simulink model "PlatoonController"  (R2018a)
settings: Solver=FixedStepDiscrete  StartTime=0.0  StopTime=2  MaxStep=0.01  RelTol=1e-4
settings Model: Creator=ATRC237_GUO  LastModifiedBy=ATRC237_GUO
settings DataIOCC: LimitDataPoints=on  SaveOutput=off  SaveTime=off
settings OptimizationCC: DefaultParameterBehavior=Inlined  UseDivisionForNetSlopeComputation=on  UseFloatMulNetSlope=on  InlineInvariantSignals=on  PassReuseOutputArgsAs=Individual arguments  ExpressionDepthLimit=2147483647  ZeroExternalMemoryAtStartup=off  ZeroInternalMemoryAtStartup=off  NoFixptDivByZeroProtection=on  EfficientFloat2IntCast=on  LifeSpan=1  OptimizeBlockOrder=speed  DifferentSizesBufferReuse=on
settings DebuggingCC: UnderspecifiedInitializationDetection=Classic  MergeDetectMultiDrivingBlocksExec=none  ParameterTunabilityLossMsg=error  FcnCallInpInsideContextMsg=warning  AllowSymbolicDim=off  StateNameClashWarn=warning  SFUnexpectedBacktrackingDiag=warning  SFNoUnconditionalDefaultTransitionDiag=warning  SFExecutionAtInitializationDiag=none
settings HardwareCC: ProdLongLongMode=on
settings SFSimCC: MATLABDynamicMemAlloc=off
settings RTWCC: SystemTargetFile=ert.tlc  TemplateMakefile=ert_default_tmf  GenerateReport=on  IncludeHyperlinkInReport=on  LaunchReport=on  TargetLang=C++  GenerateTraceInfo=on  GenerateTraceReport=on  GenerateTraceReportSl=on  GenerateTraceReportSf=on  GenerateTraceReportEml=on
settings CodeAppCC: ForceParamTrailComments=on  IgnoreCustomStorageClasses=off  OperatorAnnotations=on  SimulinkDataObjDesc=on  SFDataObjDesc=on  CustomSymbolStrGlobalVar=rt$N$M  CustomSymbolStrType=$N$M  CustomSymbolStrFcn=$N$M$F  CustomSymbolStrMacro=$N$M  InsertBlockDesc=on
settings ERTTargetCC: TargetLangStandard=C++03 (ISO)  GenerateSampleERTMain=on  IncludeMdlTerminateFcn=off  CombineSignalStateStructs=on  MultiInstanceERTCode=on  CodeInterfacePackaging=C++ class  SupportComplex=off  SupportContinuousTime=on  InlinedParameterPlacement=NonHierarchical  RootIOFormat=Structure reference  ERTCustomFileTemplate=example_file_process.tlc  ERTFilePackagingFormat=CompactWithDataFile

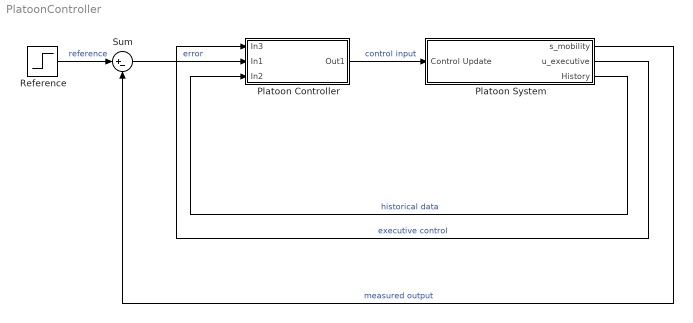
== system PlatoonController ==
  Platoon Controller : Subsystem
  Platoon System : Subsystem
  Reference : Step  SampleTime=0
  Sum : Sum  Inputs=|+-
  wires:
  Reference/1 -> Sum/1  "reference"
  Platoon System/1(s_mobility) -> Sum/2  "measured output"
  Platoon Controller/1(Out1) -> Platoon System/1(Control Update)  "control input"
  Platoon System/3(History) -> Platoon Controller/3(In2)  "historical data"
  Sum/1 -> Platoon Controller/2(In1)  "error"
  Platoon System/2(u_executive) -> Platoon Controller/1(In3)  "executive control"

== system PlatoonController/Platoon Controller ==
  In3 : Inport
  In1 : Inport  Port=2
  In2 : Inport  Port=3
  HLC : Subsystem
  LLC : Subsystem
  PLC : Subsystem
  Out1 : Outport
  wires:
  HLC/1(Out1) -> LLC/1(In1)
  PLC/1(Out1) -> HLC/1(In1)
  In1/1 -> PLC/2(Current)
  LLC/1(Out1) -> Out1/1
  In2/1 -> PLC/3(History)
  In3/1 -> PLC/1(Executive)

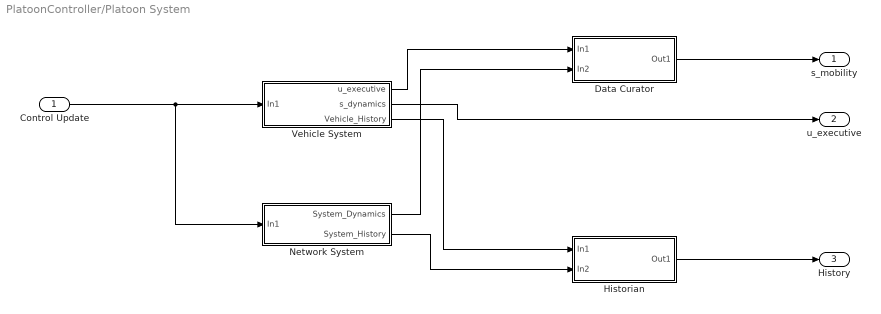
== system PlatoonController/Platoon System ==
  Control Update : Inport
  Data Curator : Subsystem
  Historian : Subsystem
  Network System : Subsystem
  Vehicle System : Subsystem
  s_mobility : Outport
  u_executive : Outport  Port=2
  History : Outport  Port=3
  wires:
  Control Update/1 -> Network System/1(In1), Vehicle System/1(In1)
  Historian/1(Out1) -> History/1
  Data Curator/1(Out1) -> s_mobility/1
  Vehicle System/1(u_executive) -> Data Curator/1(In1)
  Vehicle System/3(Vehicle_History) -> Historian/1(In1)
  Network System/1(System_Dynamics) -> Data Curator/2(In2)
  Network System/2(System_History) -> Historian/2(In2)
  Vehicle System/2(s_dynamics) -> u_executive/1

== system PlatoonController/Platoon Controller/HLC ==
  In1 : Inport
  Lateral Control : Subsystem
  Longitudinal Control : Subsystem
  Maneuver Converter : Subsystem
  Vector Concatenate : Concatenate
  Out1 : Outport
  wires:
  Longitudinal Control/1("u_accel ") -> Vector Concatenate/1
  Vector Concatenate/1 -> Out1/1
  Lateral Control/1(u_steer) -> Vector Concatenate/2
  In1/1 -> Maneuver Converter/1(In1)
  Maneuver Converter/1(Out1) -> Longitudinal Control/1(In1)
  Maneuver Converter/2(Out2) -> Lateral Control/1(In1)

== system PlatoonController/Platoon Controller/LLC ==
  In1 : Inport
  Brake : Subsystem
  Output State : Subsystem
  Steering Wheel : Subsystem
  Throttle : Subsystem
  Out1 : Outport
  wires:
  In1/1 -> Throttle/1(In1), Brake/1(In1), Steering Wheel/1(In1)
  Output State/1(Out1) -> Out1/1
  Throttle/1(Out1) -> Output State/1(In3)
  Brake/1(Out1) -> Output State/2(In1)
  Steering Wheel/1(Out1) -> Output State/3(In2)

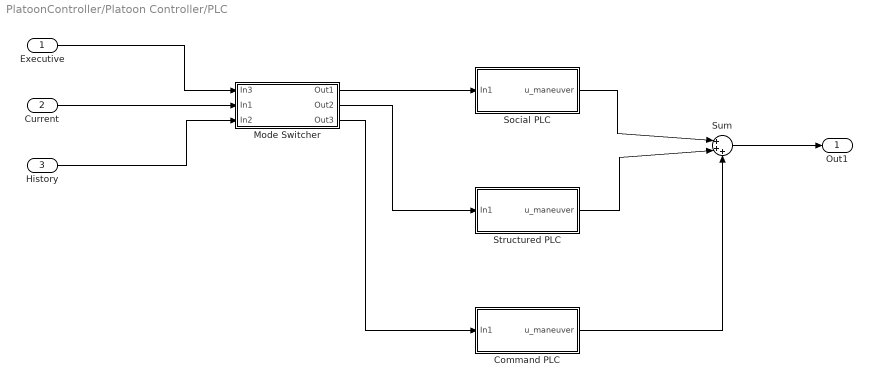
== system PlatoonController/Platoon Controller/PLC ==
  Executive : Inport
  Current : Inport  Port=2
  History : Inport  Port=3
  Command PLC : Subsystem
  Mode Switcher : Subsystem
  Social PLC : Subsystem
  Structured PLC : Subsystem
  Sum : Sum  Inputs=|+++
  Out1 : Outport
  wires:
  Current/1 -> Mode Switcher/2(In1)
  Mode Switcher/1(Out1) -> Social PLC/1(In1)
  Mode Switcher/2(Out2) -> Structured PLC/1(In1)
  Social PLC/1(u_maneuver) -> Sum/1
  Structured PLC/1(u_maneuver) -> Sum/2
  Sum/1 -> Out1/1
  History/1 -> Mode Switcher/3(In2)
  Executive/1 -> Mode Switcher/1(In3)
  Command PLC/1(u_maneuver) -> Sum/3
  Mode Switcher/3(Out3) -> Command PLC/1(In1)

== system PlatoonController/Platoon System/Data Curator ==
  In1 : Inport
  In2 : Inport  Port=2
  Vector Concatenate : Concatenate
  Out1 : Outport
  wires:
  In2/1 -> Vector Concatenate/2
  In1/1 -> Vector Concatenate/1
  Vector Concatenate/1 -> Out1/1

== system PlatoonController/Platoon System/Historian ==
  In1 : Inport
  In2 : Inport  Port=2
  Vector Concatenate : Concatenate
  Out1 : Outport
  wires:
  In1/1 -> Vector Concatenate/1
  In2/1 -> Vector Concatenate/2
  Vector Concatenate/1 -> Out1/1

== system PlatoonController/Platoon System/Network System ==
  In1 : Inport
  CAV Network System : Subsystem
  Communication System : Subsystem
  Storage System : Subsystem
  System_Dynamics : Outport
  System_History : Outport  Port=2
  wires:
  Communication System/1(Out1) -> CAV Network System/1(In1)
  CAV Network System/1(Out1) -> System_Dynamics/1, Storage System/1(In1)
  In1/1 -> Communication System/1(In1)
  Storage System/1(Out1) -> System_History/1

== system PlatoonController/Platoon System/Vehicle System ==
  In1 : Inport
  CAV System : Subsystem
  Storage System : Subsystem
  u_executive : Outport
  s_dynamics : Outport  Port=2
  Vehicle_History : Outport  Port=3
  wires:
  In1/1 -> Storage System/1(In1), CAV System/1(In1)
  CAV System/1(u_executive) -> u_executive/1
  Storage System/1(Out1) -> Vehicle_History/1
  CAV System/2(s_dynamics) -> s_dynamics/1

== system PlatoonController/Platoon Controller/HLC/Lateral Control ==
  In1 : Inport
  "Steer " : Subsystem
  u_steer : Outport
  wires:
  In1/1 -> "Steer "/1(In1)
  "Steer "/1(Out1) -> u_steer/1

== system PlatoonController/Platoon Controller/HLC/Longitudinal Control ==
  In1 : Inport
  Acceleration : Subsystem
  Brake : Subsystem
  Throttle : Subsystem
  "u_accel " : Outport
  wires:
  Throttle/1(Out1) -> Acceleration/1(In1)
  Brake/1(Out1) -> Acceleration/2(In2)
  Acceleration/1(Out1) -> "u_accel "/1
  In1/1 -> Brake/1(In1), Throttle/1(In1)

== system PlatoonController/Platoon Controller/HLC/Maneuver Converter ==
  In1 : Inport
  Out1 : Outport
  Out2 : Outport  Port=2
  wires:
  In1/1 -> Out1/1

== system PlatoonController/Platoon Controller/LLC/Brake ==
  In1 : Inport
  Out1 : Outport
  wires:
  In1/1 -> Out1/1

== system PlatoonController/Platoon Controller/LLC/Output State ==
  In3 : Inport
  In1 : Inport  Port=2
  In2 : Inport  Port=3
  Out1 : Outport
  wires:
  In1/1 -> Out1/1

== system PlatoonController/Platoon Controller/LLC/Steering Wheel ==
  In1 : Inport
  Out1 : Outport
  wires:
  In1/1 -> Out1/1

== system PlatoonController/Platoon Controller/LLC/Throttle ==
  In1 : Inport
  Out1 : Outport
  wires:
  In1/1 -> Out1/1

== system PlatoonController/Platoon Controller/PLC/Command PLC ==
  In1 : Inport
  Maneuver Calculator : Subsystem
  Predictor : Subsystem
  Recognizer : Subsystem
  Sustainer : Subsystem
  Vector Concatenate : Concatenate
  u_maneuver : Outport
  wires:
  Sustainer/1(Out1) -> Maneuver Calculator/1(In1), Predictor/1(In1)
  Recognizer/1(Out1) -> Vector Concatenate/1, Sustainer/1(In1)
  Predictor/1(Out1) -> Maneuver Calculator/2(In2)
  Maneuver Calculator/1(Maneuver_Coefficient) -> Vector Concatenate/2
  In1/1 -> Recognizer/1(In1)
  Vector Concatenate/1 -> u_maneuver/1

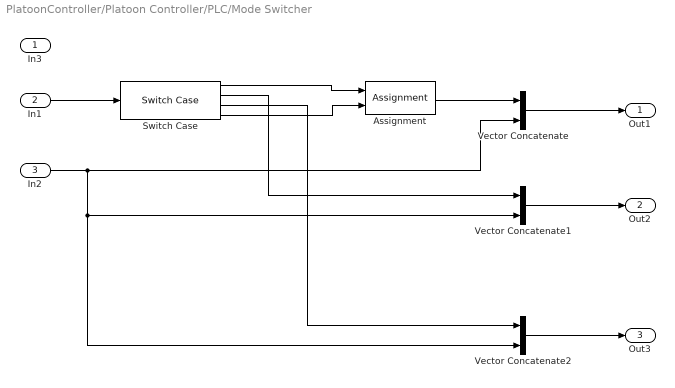
== system PlatoonController/Platoon Controller/PLC/Mode Switcher ==
  In3 : Inport
  In1 : Inport  Port=2
  In2 : Inport  Port=3
  Assignment : Assignment  DiagnosticForDimensions=Warning  IndexOptions=Index vector (dialog)  Indices=1  OutputSizes=1
  Switch Case : SwitchCase  CaseConditions={1, 2, 3}
  Vector Concatenate : Concatenate
  Vector Concatenate1 : Concatenate
  Vector Concatenate2 : Concatenate
  Out1 : Outport
  Out2 : Outport  Port=2
  Out3 : Outport  Port=3
  wires:
  In1/1 -> Switch Case/1
  Switch Case/1 -> Assignment/1
  Switch Case/4 -> Assignment/2
  Vector Concatenate1/1 -> Out2/1
  Assignment/1 -> Vector Concatenate/1
  Switch Case/2 -> Vector Concatenate1/1
  Vector Concatenate/1 -> Out1/1
  Vector Concatenate2/1 -> Out3/1
  In2/1 -> Vector Concatenate/2, Vector Concatenate2/2, Vector Concatenate1/2
  Switch Case/3 -> Vector Concatenate2/1

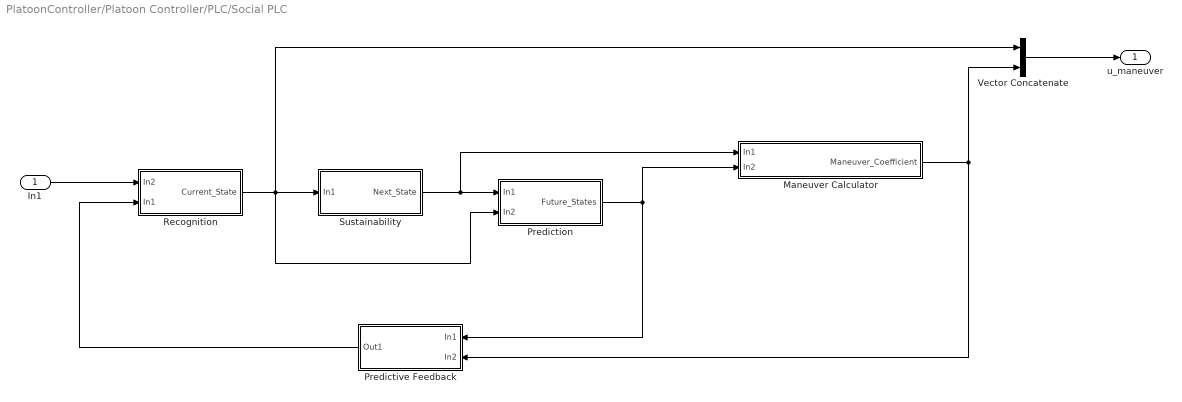
== system PlatoonController/Platoon Controller/PLC/Social PLC ==
  In1 : Inport
  Maneuver Calculator : Subsystem
  Prediction : Subsystem
  Predictive Feedback : Subsystem
  Recognition : Subsystem
  Sustainability : Subsystem
  Vector Concatenate : Concatenate
  u_maneuver : Outport
  wires:
  Prediction/1(Future_States) -> Maneuver Calculator/2(In2), Predictive Feedback/1(In1)
  In1/1 -> Recognition/1(In2)
  Sustainability/1(Next_State) -> Maneuver Calculator/1(In1), Prediction/1(In1)
  Recognition/1(Current_State) -> Vector Concatenate/1, Prediction/2(In2), Sustainability/1(In1)
  Maneuver Calculator/1(Maneuver_Coefficient) -> Vector Concatenate/2, Predictive Feedback/2(In2)
  Predictive Feedback/1(Out1) -> Recognition/2(In1)
  Vector Concatenate/1 -> u_maneuver/1

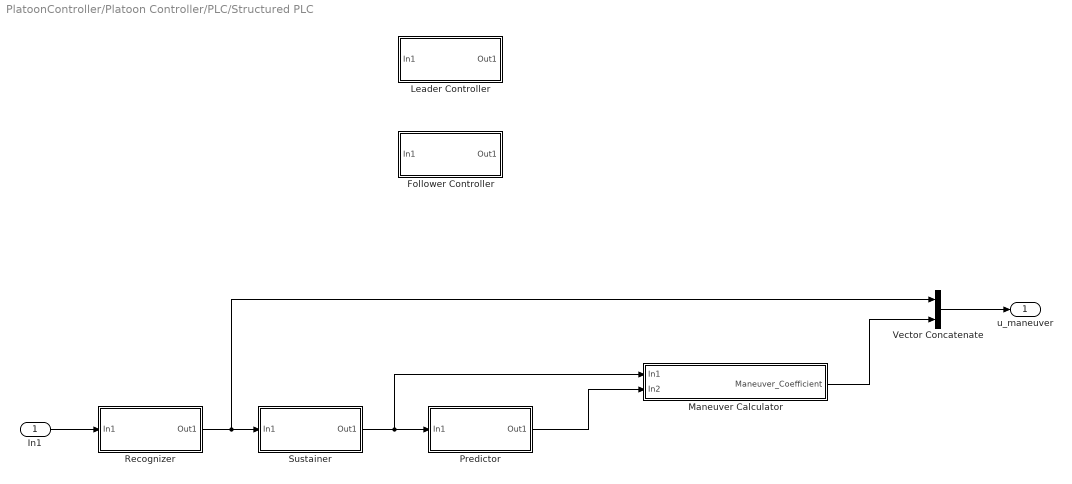
== system PlatoonController/Platoon Controller/PLC/Structured PLC ==
  In1 : Inport
  Follower Controller : Subsystem
  Leader Controller : Subsystem
  Maneuver Calculator : Subsystem
  Predictor : Subsystem
  Recognizer : Subsystem
  Sustainer : Subsystem
  Vector Concatenate : Concatenate
  u_maneuver : Outport
  wires:
  Sustainer/1(Out1) -> Maneuver Calculator/1(In1), Predictor/1(In1)
  Recognizer/1(Out1) -> Vector Concatenate/1, Sustainer/1(In1)
  Predictor/1(Out1) -> Maneuver Calculator/2(In2)
  Maneuver Calculator/1(Maneuver_Coefficient) -> Vector Concatenate/2
  In1/1 -> Recognizer/1(In1)
  Vector Concatenate/1 -> u_maneuver/1

== system PlatoonController/Platoon System/Network System/CAV Network System ==
  In1 : Inport
  Out1 : Outport
  wires:
  In1/1 -> Out1/1

== system PlatoonController/Platoon System/Network System/Communication System ==
  In1 : Inport
  Out1 : Outport
  wires:
  In1/1 -> Out1/1

== system PlatoonController/Platoon System/Network System/Storage System ==
  In1 : Inport
  Out1 : Outport
  wires:
  In1/1 -> Out1/1

== system PlatoonController/Platoon System/Vehicle System/CAV System ==
  In1 : Inport
  AVCB : Subsystem
  Vehicle Dynamics : Subsystem
  u_executive : Outport
  s_dynamics : Outport  Port=2
  wires:
  In1/1 -> AVCB/1(In1), Vehicle Dynamics/1(In1)
  AVCB/1(Out1) -> u_executive/1
  Vehicle Dynamics/1(Out1) -> s_dynamics/1

== system PlatoonController/Platoon System/Vehicle System/Storage System ==
  In1 : Inport
  Out1 : Outport
  wires:
  In1/1 -> Out1/1

== system PlatoonController/Platoon Controller/HLC/Lateral Control/Steer  ==
  In1 : Inport
  Out1 : Outport
  wires:
  In1/1 -> Out1/1

== system PlatoonController/Platoon Controller/HLC/Longitudinal Control/Acceleration ==
  In1 : Inport
  In2 : Inport  Port=2
  Out1 : Outport
  wires:
  In1/1 -> Out1/1

== system PlatoonController/Platoon Controller/HLC/Longitudinal Control/Brake ==
  In1 : Inport
  Out1 : Outport
  wires:
  In1/1 -> Out1/1

== system PlatoonController/Platoon Controller/HLC/Longitudinal Control/Throttle ==
  In1 : Inport
  Out1 : Outport
  wires:
  In1/1 -> Out1/1

== system PlatoonController/Platoon Controller/PLC/Command PLC/Maneuver Calculator ==
  In1 : Inport
  In2 : Inport  Port=2
  Sum : Sum  Inputs=|++
  Maneuver_Coefficient : Outport
  wires:
  In2/1 -> Sum/1
  In1/1 -> Sum/2
  Sum/1 -> Maneuver_Coefficient/1

== system PlatoonController/Platoon Controller/PLC/Command PLC/Predictor ==
  In1 : Inport
  Out1 : Outport
  wires:
  In1/1 -> Out1/1

== system PlatoonController/Platoon Controller/PLC/Command PLC/Recognizer ==
  In1 : Inport
  Out1 : Outport
  wires:
  In1/1 -> Out1/1

== system PlatoonController/Platoon Controller/PLC/Command PLC/Sustainer ==
  In1 : Inport
  Out1 : Outport
  wires:
  In1/1 -> Out1/1

== system PlatoonController/Platoon Controller/PLC/Social PLC/Maneuver Calculator ==
  In1 : Inport
  In2 : Inport  Port=2
  Sum : Sum  Inputs=|++
  Maneuver_Coefficient : Outport
  wires:
  In2/1 -> Sum/1
  In1/1 -> Sum/2
  Sum/1 -> Maneuver_Coefficient/1

== system PlatoonController/Platoon Controller/PLC/Social PLC/Prediction ==
  In1 : Inport
  In2 : Inport  Port=2
  Predictor : Subsystem
  Future_States : Outport
  wires:
  In1/1 -> Predictor/1(In1)
  Predictor/1(Out1) -> Future_States/1
  In2/1 -> Predictor/2(In2)

== system PlatoonController/Platoon Controller/PLC/Social PLC/Predictive Feedback ==
  In1 : Inport
  In2 : Inport  Port=2
  Vector Concatenate : Concatenate
  Out1 : Outport
  wires:
  In2/1 -> Vector Concatenate/2
  In1/1 -> Vector Concatenate/1
  Vector Concatenate/1 -> Out1/1

== system PlatoonController/Platoon Controller/PLC/Social PLC/Recognition ==
  In2 : Inport
  In1 : Inport  Port=2
  Estimator : Subsystem
  Refiner : Subsystem
  Current_State : Outport
  wires:
  In2/1 -> Estimator/1(In1)
  In1/1 -> Refiner/2(In2)
  Estimator/1(Out1) -> Refiner/1(In1)
  Refiner/1(Out1) -> Current_State/1

== system PlatoonController/Platoon Controller/PLC/Social PLC/Sustainability ==
  In1 : Inport
  Negotiator : Subsystem
  Optimizer : Subsystem
  Next_State : Outport
  wires:
  Optimizer/3(u_vehicle) -> Negotiator/3(In3)
  Optimizer/1(u_crowd) -> Negotiator/1(In1)
  Optimizer/2(u_safety) -> Negotiator/2(In2)
  In1/1 -> Optimizer/1(In1)
  Negotiator/1(Out1) -> Next_State/1

== system PlatoonController/Platoon Controller/PLC/Structured PLC/Follower Controller ==
  In1 : Inport
  Out1 : Outport
  wires:
  In1/1 -> Out1/1

== system PlatoonController/Platoon Controller/PLC/Structured PLC/Leader Controller ==
  In1 : Inport
  Out1 : Outport
  wires:
  In1/1 -> Out1/1

== system PlatoonController/Platoon Controller/PLC/Structured PLC/Maneuver Calculator ==
  In1 : Inport
  In2 : Inport  Port=2
  Sum : Sum  Inputs=|++
  Maneuver_Coefficient : Outport
  wires:
  In2/1 -> Sum/1
  In1/1 -> Sum/2
  Sum/1 -> Maneuver_Coefficient/1

== system PlatoonController/Platoon Controller/PLC/Structured PLC/Predictor ==
  In1 : Inport
  Out1 : Outport
  wires:
  In1/1 -> Out1/1

== system PlatoonController/Platoon Controller/PLC/Structured PLC/Recognizer ==
  In1 : Inport
  Out1 : Outport
  wires:
  In1/1 -> Out1/1

== system PlatoonController/Platoon Controller/PLC/Structured PLC/Sustainer ==
  In1 : Inport
  Out1 : Outport
  wires:
  In1/1 -> Out1/1

== system PlatoonController/Platoon System/Vehicle System/CAV System/AVCB ==
  In1 : Inport
  Out1 : Outport
  wires:
  In1/1 -> Out1/1

== system PlatoonController/Platoon System/Vehicle System/CAV System/Vehicle Dynamics ==
  In1 : Inport
  Out1 : Outport
  wires:
  In1/1 -> Out1/1

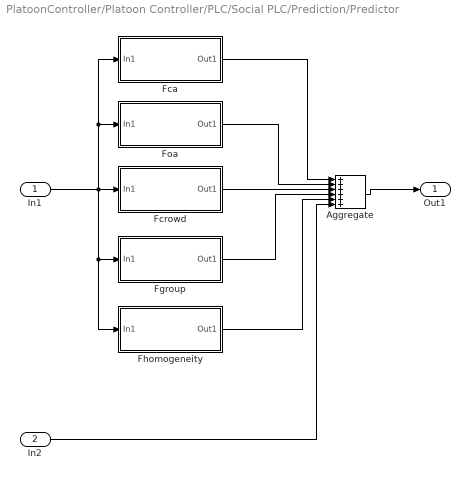
== system PlatoonController/Platoon Controller/PLC/Social PLC/Prediction/Predictor ==
  In1 : Inport
  In2 : Inport  Port=2
  Aggregate : Sum  Inputs=++++++
  Fca : Subsystem
  Fcrowd : Subsystem
  Fgroup : Subsystem
  Fhomogeneity : Subsystem
  Foa : Subsystem
  Out1 : Outport
  wires:
  In1/1 -> Fhomogeneity/1(In1), Fgroup/1(In1), Fca/1(In1), Foa/1(In1), Fcrowd/1(In1)
  Fca/1(Out1) -> Aggregate/1
  Aggregate/1 -> Out1/1
  Foa/1(Out1) -> Aggregate/2
  Fcrowd/1(Out1) -> Aggregate/3
  Fgroup/1(Out1) -> Aggregate/4
  Fhomogeneity/1(Out1) -> Aggregate/5
  In2/1 -> Aggregate/6

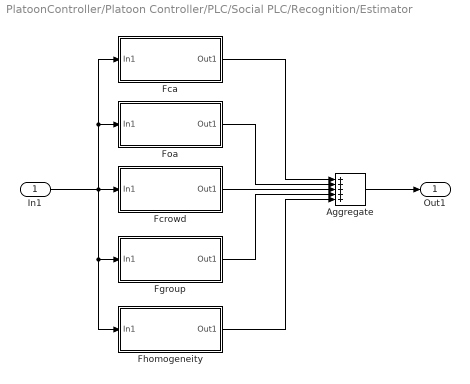
== system PlatoonController/Platoon Controller/PLC/Social PLC/Recognition/Estimator ==
  In1 : Inport
  Aggregate : Sum  Inputs=+++++
  Fca : Subsystem
  Fcrowd : Subsystem
  Fgroup : Subsystem
  Fhomogeneity : Subsystem
  Foa : Subsystem
  Out1 : Outport
  wires:
  In1/1 -> Fhomogeneity/1(In1), Fgroup/1(In1), Fca/1(In1), Foa/1(In1), Fcrowd/1(In1)
  Fca/1(Out1) -> Aggregate/1
  Aggregate/1 -> Out1/1
  Foa/1(Out1) -> Aggregate/2
  Fcrowd/1(Out1) -> Aggregate/3
  Fgroup/1(Out1) -> Aggregate/4
  Fhomogeneity/1(Out1) -> Aggregate/5

== system PlatoonController/Platoon Controller/PLC/Social PLC/Recognition/Refiner ==
  In1 : Inport
  In2 : Inport  Port=2
  Sum of Elements : Sum
  Out1 : Outport
  wires:
  In1/1 -> Sum of Elements/1
  In2/1 -> Sum of Elements/2
  Sum of Elements/1 -> Out1/1

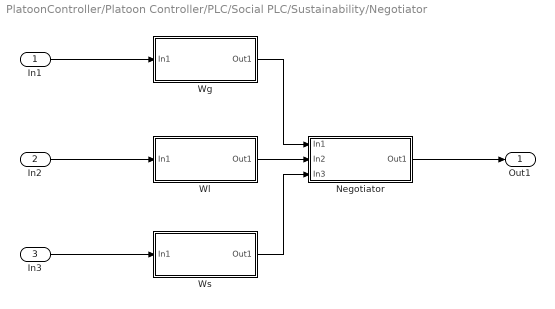
== system PlatoonController/Platoon Controller/PLC/Social PLC/Sustainability/Negotiator ==
  In1 : Inport
  In2 : Inport  Port=2
  In3 : Inport  Port=3
  Negotiator : Subsystem
  Wg : Subsystem
  Wl : Subsystem
  Ws : Subsystem
  Out1 : Outport
  wires:
  Negotiator/1(Out1) -> Out1/1
  In1/1 -> Wg/1(In1)
  In2/1 -> Wl/1(In1)
  In3/1 -> Ws/1(In1)
  Wg/1(Out1) -> Negotiator/1(In1)
  Wl/1(Out1) -> Negotiator/2(In2)
  Ws/1(Out1) -> Negotiator/3(In3)

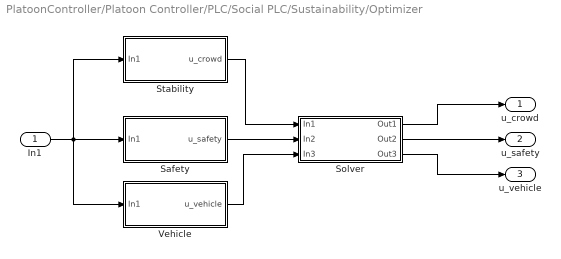
== system PlatoonController/Platoon Controller/PLC/Social PLC/Sustainability/Optimizer ==
  In1 : Inport
  Safety : Subsystem
  Solver : Subsystem
  Stability : Subsystem
  Vehicle : Subsystem
  u_crowd : Outport
  u_safety : Outport  Port=2
  u_vehicle : Outport  Port=3
  wires:
  In1/1 -> Stability/1(In1), Vehicle/1(In1), Safety/1(In1)
  Solver/3(Out3) -> u_vehicle/1
  Vehicle/1(u_vehicle) -> Solver/3(In3)
  Safety/1(u_safety) -> Solver/2(In2)
  Stability/1(u_crowd) -> Solver/1(In1)
  Solver/2(Out2) -> u_safety/1
  Solver/1(Out1) -> u_crowd/1

== system PlatoonController/Platoon Controller/PLC/Social PLC/Prediction/Predictor/Fca ==
  In1 : Inport
  Gain : Gain
  Out1 : Outport
  wires:
  Gain/1 -> Out1/1
  In1/1 -> Gain/1

== system PlatoonController/Platoon Controller/PLC/Social PLC/Prediction/Predictor/Fcrowd ==
  In1 : Inport
  Gain : Gain
  Out1 : Outport
  wires:
  Gain/1 -> Out1/1
  In1/1 -> Gain/1

== system PlatoonController/Platoon Controller/PLC/Social PLC/Prediction/Predictor/Fgroup ==
  In1 : Inport
  Gain : Gain
  Out1 : Outport
  wires:
  Gain/1 -> Out1/1
  In1/1 -> Gain/1

== system PlatoonController/Platoon Controller/PLC/Social PLC/Prediction/Predictor/Fhomogeneity ==
  In1 : Inport
  Gain : Gain
  Out1 : Outport
  wires:
  Gain/1 -> Out1/1
  In1/1 -> Gain/1

== system PlatoonController/Platoon Controller/PLC/Social PLC/Prediction/Predictor/Foa ==
  In1 : Inport
  Gain : Gain
  Out1 : Outport
  wires:
  Gain/1 -> Out1/1
  In1/1 -> Gain/1

== system PlatoonController/Platoon Controller/PLC/Social PLC/Recognition/Estimator/Fca ==
  In1 : Inport
  Gain : Gain
  Out1 : Outport
  wires:
  Gain/1 -> Out1/1
  In1/1 -> Gain/1

== system PlatoonController/Platoon Controller/PLC/Social PLC/Recognition/Estimator/Fcrowd ==
  In1 : Inport
  Gain : Gain
  Out1 : Outport
  wires:
  Gain/1 -> Out1/1
  In1/1 -> Gain/1

== system PlatoonController/Platoon Controller/PLC/Social PLC/Recognition/Estimator/Fgroup ==
  In1 : Inport
  Gain : Gain
  Out1 : Outport
  wires:
  Gain/1 -> Out1/1
  In1/1 -> Gain/1

== system PlatoonController/Platoon Controller/PLC/Social PLC/Recognition/Estimator/Fhomogeneity ==
  In1 : Inport
  Gain : Gain
  Out1 : Outport
  wires:
  Gain/1 -> Out1/1
  In1/1 -> Gain/1

== system PlatoonController/Platoon Controller/PLC/Social PLC/Recognition/Estimator/Foa ==
  In1 : Inport
  Gain : Gain
  Out1 : Outport
  wires:
  Gain/1 -> Out1/1
  In1/1 -> Gain/1

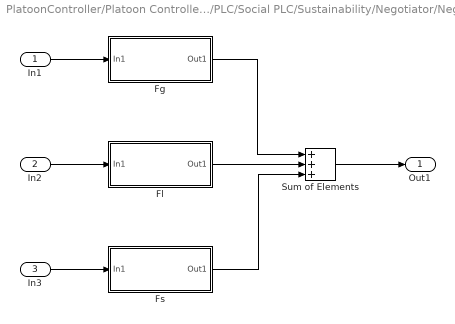
== system PlatoonController/Platoon Controller/PLC/Social PLC/Sustainability/Negotiator/Negotiator ==
  In1 : Inport
  In2 : Inport  Port=2
  In3 : Inport  Port=3
  Fg : Subsystem
  Fl : Subsystem
  Fs : Subsystem
  Sum of Elements : Sum  Inputs=+++
  Out1 : Outport
  wires:
  Sum of Elements/1 -> Out1/1
  In1/1 -> Fg/1(In1)
  In2/1 -> Fl/1(In1)
  In3/1 -> Fs/1(In1)
  Fg/1(Out1) -> Sum of Elements/1
  Fl/1(Out1) -> Sum of Elements/2
  Fs/1(Out1) -> Sum of Elements/3

== system PlatoonController/Platoon Controller/PLC/Social PLC/Sustainability/Negotiator/Wg ==
  In1 : Inport
  Out1 : Outport
  wires:
  In1/1 -> Out1/1

== system PlatoonController/Platoon Controller/PLC/Social PLC/Sustainability/Negotiator/Wl ==
  In1 : Inport
  Out1 : Outport
  wires:
  In1/1 -> Out1/1

== system PlatoonController/Platoon Controller/PLC/Social PLC/Sustainability/Negotiator/Ws ==
  In1 : Inport
  Out1 : Outport
  wires:
  In1/1 -> Out1/1

== system PlatoonController/Platoon Controller/PLC/Social PLC/Sustainability/Optimizer/Safety ==
  In1 : Inport
  Adversary : Subsystem
  Danger : Subsystem
  Solver : Subsystem
  u_safety : Outport
  wires:
  Adversary/1(Out1) -> Solver/1(In1)
  Solver/1(Out1) -> u_safety/1
  In1/1 -> Danger/1(In1), Adversary/1(In1)
  Danger/1(Out1) -> Solver/2(In2)

== system PlatoonController/Platoon Controller/PLC/Social PLC/Sustainability/Optimizer/Solver ==
  In1 : Inport
  In2 : Inport  Port=2
  In3 : Inport  Port=3
  Out1 : Outport
  Out2 : Outport  Port=2
  Out3 : Outport  Port=3
  wires:
  In1/1 -> Out1/1
  In2/1 -> Out2/1
  In3/1 -> Out3/1

== system PlatoonController/Platoon Controller/PLC/Social PLC/Sustainability/Optimizer/Stability ==
  In1 : Inport
  Flock : Subsystem
  Solver : Subsystem
  Stabilize : Subsystem
  u_crowd : Outport
  wires:
  In1/1 -> Flock/1(In1), Stabilize/1(In1)
  Solver/1(Out1) -> u_crowd/1
  Flock/1(Out1) -> Solver/1(In1)
  Stabilize/1(Out1) -> Solver/2(In2)

== system PlatoonController/Platoon Controller/PLC/Social PLC/Sustainability/Optimizer/Vehicle ==
  In1 : Inport
  Interests : Subsystem
  Solver : Subsystem
  Survival : Subsystem
  u_vehicle : Outport
  wires:
  In1/1 -> Survival/1(In1), Interests/1(In1)
  Solver/1(Out1) -> u_vehicle/1
  Interests/1(Out1) -> Solver/2(In2)
  Survival/1(Out1) -> Solver/1(In1)

== system PlatoonController/Platoon Controller/PLC/Social PLC/Sustainability/Negotiator/Negotiator/Fg ==
  In1 : Inport
  Out1 : Outport
  wires:
  In1/1 -> Out1/1

== system PlatoonController/Platoon Controller/PLC/Social PLC/Sustainability/Negotiator/Negotiator/Fl ==
  In1 : Inport
  Out1 : Outport
  wires:
  In1/1 -> Out1/1

== system PlatoonController/Platoon Controller/PLC/Social PLC/Sustainability/Negotiator/Negotiator/Fs ==
  In1 : Inport
  Out1 : Outport
  wires:
  In1/1 -> Out1/1

== system PlatoonController/Platoon Controller/PLC/Social PLC/Sustainability/Optimizer/Safety/Adversary ==
  In1 : Inport
  Out1 : Outport
  wires:
  In1/1 -> Out1/1

== system PlatoonController/Platoon Controller/PLC/Social PLC/Sustainability/Optimizer/Safety/Danger ==
  In1 : Inport
  Out1 : Outport
  wires:
  In1/1 -> Out1/1

== system PlatoonController/Platoon Controller/PLC/Social PLC/Sustainability/Optimizer/Safety/Solver ==
  In1 : Inport
  In2 : Inport  Port=2
  Out1 : Outport
  wires:
  In1/1 -> Out1/1

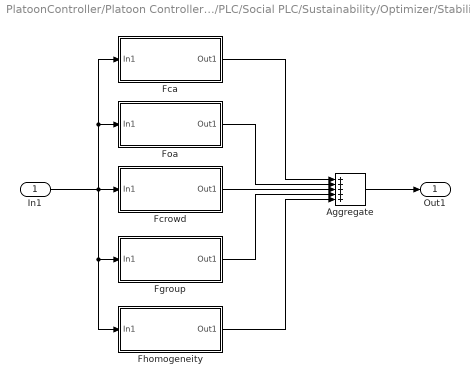
== system PlatoonController/Platoon Controller/PLC/Social PLC/Sustainability/Optimizer/Stability/Flock ==
  In1 : Inport
  Aggregate : Sum  Inputs=+++++
  Fca : Subsystem
  Fcrowd : Subsystem
  Fgroup : Subsystem
  Fhomogeneity : Subsystem
  Foa : Subsystem
  Out1 : Outport
  wires:
  In1/1 -> Fhomogeneity/1(In1), Fgroup/1(In1), Fca/1(In1), Foa/1(In1), Fcrowd/1(In1)
  Fca/1(Out1) -> Aggregate/1
  Aggregate/1 -> Out1/1
  Foa/1(Out1) -> Aggregate/2
  Fcrowd/1(Out1) -> Aggregate/3
  Fgroup/1(Out1) -> Aggregate/4
  Fhomogeneity/1(Out1) -> Aggregate/5

== system PlatoonController/Platoon Controller/PLC/Social PLC/Sustainability/Optimizer/Stability/Solver ==
  In1 : Inport
  In2 : Inport  Port=2
  Out1 : Outport
  wires:
  In1/1 -> Out1/1

== system PlatoonController/Platoon Controller/PLC/Social PLC/Sustainability/Optimizer/Stability/Stabilize ==
  In1 : Inport
  Aggregator : Sum
  Regulation : Subsystem
  Stability : Subsystem
  Out1 : Outport
  wires:
  Aggregator/1 -> Out1/1
  Stability/1(Out1) -> Aggregator/1
  Regulation/1(Out1) -> Aggregator/2
  In1/1 -> Regulation/1(In1), Stability/1(In1)

== system PlatoonController/Platoon Controller/PLC/Social PLC/Sustainability/Optimizer/Vehicle/Interests ==
  In1 : Inport
  Out1 : Outport
  wires:
  In1/1 -> Out1/1

== system PlatoonController/Platoon Controller/PLC/Social PLC/Sustainability/Optimizer/Vehicle/Solver ==
  In1 : Inport
  In2 : Inport  Port=2
  Out1 : Outport
  wires:
  In1/1 -> Out1/1

== system PlatoonController/Platoon Controller/PLC/Social PLC/Sustainability/Optimizer/Vehicle/Survival ==
  In1 : Inport
  Out1 : Outport
  wires:
  In1/1 -> Out1/1

== system PlatoonController/Platoon Controller/PLC/Social PLC/Sustainability/Optimizer/Stability/Flock/Fca ==
  In1 : Inport
  Gain : Gain
  Out1 : Outport
  wires:
  Gain/1 -> Out1/1
  In1/1 -> Gain/1

== system PlatoonController/Platoon Controller/PLC/Social PLC/Sustainability/Optimizer/Stability/Flock/Fcrowd ==
  In1 : Inport
  Gain : Gain
  Out1 : Outport
  wires:
  Gain/1 -> Out1/1
  In1/1 -> Gain/1

== system PlatoonController/Platoon Controller/PLC/Social PLC/Sustainability/Optimizer/Stability/Flock/Fgroup ==
  In1 : Inport
  Gain : Gain
  Out1 : Outport
  wires:
  Gain/1 -> Out1/1
  In1/1 -> Gain/1

== system PlatoonController/Platoon Controller/PLC/Social PLC/Sustainability/Optimizer/Stability/Flock/Fhomogeneity ==
  In1 : Inport
  Gain : Gain
  Out1 : Outport
  wires:
  Gain/1 -> Out1/1
  In1/1 -> Gain/1

== system PlatoonController/Platoon Controller/PLC/Social PLC/Sustainability/Optimizer/Stability/Flock/Foa ==
  In1 : Inport
  Gain : Gain
  Out1 : Outport
  wires:
  Gain/1 -> Out1/1
  In1/1 -> Gain/1

== system PlatoonController/Platoon Controller/PLC/Social PLC/Sustainability/Optimizer/Stability/Stabilize/Regulation ==
  In1 : Inport
  Out1 : Outport
  wires:
  In1/1 -> Out1/1

== system PlatoonController/Platoon Controller/PLC/Social PLC/Sustainability/Optimizer/Stability/Stabilize/Stability ==
  In1 : Inport
  Out1 : Outport
  wires:
  In1/1 -> Out1/1
